simulink model "Quadcopter_Flight_Control_Simulink_payload"  (R2023b)
settings: Solver=VariableStepAuto  StartTime=0.0  StopTime=50  RelTol=1e-3
values from neighbouring files (symbols this model uses):
  A_x = 0.005581    [Quadcopter_Flight_Quantities.m]    (also in Quadcopter_Flight_Quantities_2.m)
  A_y = 0.008085    [Quadcopter_Flight_Quantities.m]    (also in Quadcopter_Flight_Quantities_2.m)
  A_z = 0.022259    [Quadcopter_Flight_Quantities.m]    (also in Quadcopter_Flight_Quantities_2.m)
  air_rho = 1.225    [Quadcopter_Flight_Quantities.m]    (also in Quadcopter_Flight_Quantities_2.m)
  Cd = 37.4    [Quadcopter_Flight_Quantities.m]    (also in Quadcopter_Flight_Quantities_2.m)
  d_p = 0.24    [Quadcopter_Flight_Quantities.m]    (also in Quadcopter_Flight_Quantities_2.m)
  g = 9.81    [Quadcopter_Flight_Quantities.m]    (also in Quadcopter_Flight_Quantities_2.m)
  k_m = 2.1783E-06    (= 2.1783e-06)    [Quadcopter_Flight_Quantities.m]    (also in Quadcopter_Flight_Quantities_2.m = 1)
  k_t = 7.3070E-05    (= 7.307e-05)    [Quadcopter_Flight_Quantities.m]    (also in Quadcopter_Flight_Quantities_2.m = 1)
  m = 2.3    [Quadcopter_Flight_Quantities.m]    (also in Quadcopter_Flight_Quantities_2.m)
  m_p = 2.530    (= 2.53)    [Quadcopter_Flight_Quantities.m]    (also in Quadcopter_Flight_Quantities_2.m)
  propeller_max = 4947*((2*pi)/60)    (= 518.048628577)    [Quadcopter_Flight_Quantities.m]    (also in Quadcopter_Flight_Quantities_2.m = 10)
libraries: matrix_library x5, slpidlib x4, aerolibasang x1, aerolibanimutils x1, shared6dof x1
settings Model: Creator=matho  LastModifiedBy=umayr
settings OptimizationCC: ReuseModelBlockBuffer=off

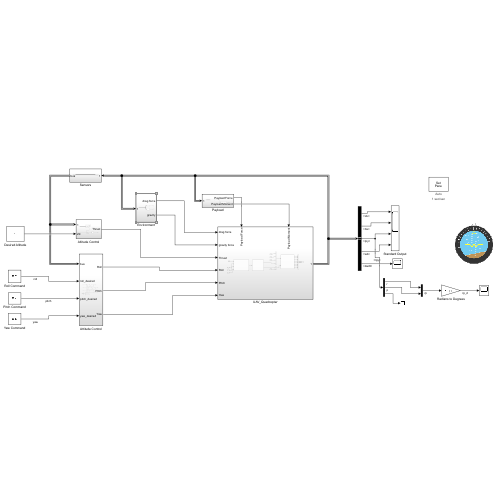
[thumbnail: Simulink's stored preview of the top-level diagram]
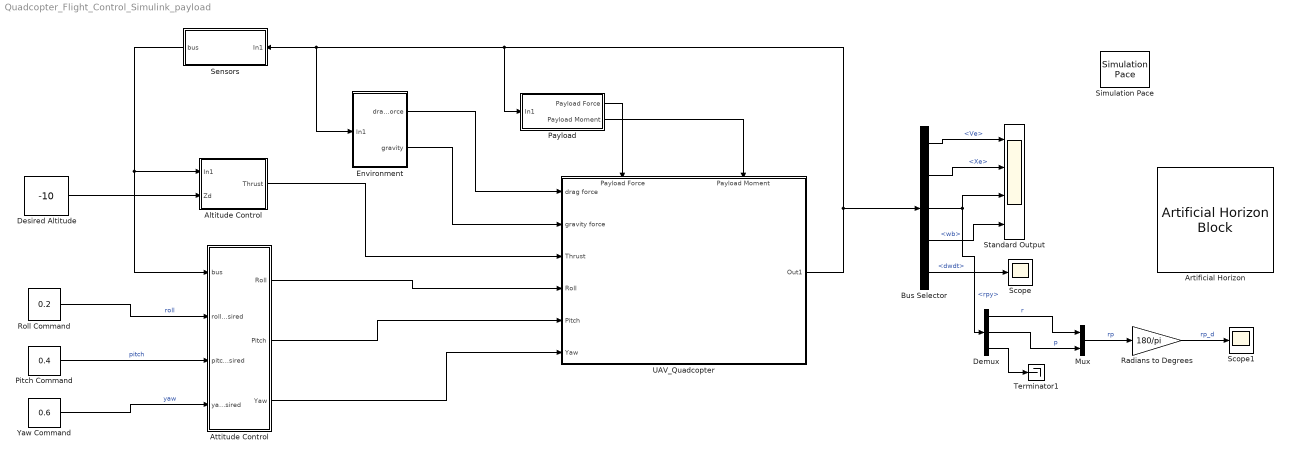
== system Quadcopter_Flight_Control_Simulink_payload ==
  Altitude Control : Subsystem
  Artificial Horizon : ArtificialHorizonBlock
  Attitude Control : Subsystem
  Bus Selector : BusSelector  OutputSignals=Ve,Xe,rpy,wb,dwdt
  Demux : Demux  Outputs=3
  Desired Altitude : Constant  Value=-10
  Environment : Subsystem
  Mux : Mux  Inputs=2
  Payload : Subsystem
  Pitch Command : Constant  Value=0.4
  Radians to Degrees : Gain  Gain=180/pi
  Roll Command : Constant  Value=0.2
  Scope : Scope
  Scope1 : Scope
  Sensors : Subsystem
  Simulation Pace : aerolibanimutils/Simulation Pace  SimulationPace=1  SleepMode=Auto  OutputPaceError=off  SampleTime=1/30
  Standard Output : Scope  NumInputPorts=4
  Terminator1 : Terminator
  UAV_Quadcopter : Subsystem
      settings: PortSchema="{\"entries\":[{\"content\":{\"sides\":[{\"content\":{\"connectorIds\":[\"In1\",\"In2\",\"In3\",\"In4\",\"In5\",\"In6\"]},\"type\":\"ConnectorPlacement.EquallySpacedRectSide\",\"uuid\":\"e9094f1d-4470-4b4b-9e27-8ba5c7ba494b\"},{\"content\":{\"connectorIds\":[\"Out1\"],\"side\":\"RIGHT\"},\"type\":\"ConnectorPlacement.EquallySpacedRectSide\",\"uuid\":\"c85a969e-3765-49d4-918f-aa5822e07523\"},{\"content\":{\"connectorIds\":[\"In7\",\"In8\"],\"side\":\"TOP\"},\"type\":\"ConnectorPlacement.EquallySpacedRectSide\",\"uuid\":\"755ec0fa-64b0-46e0-b496-7abb4caa3b84\"}]},\"type\":\"ConnectorPlacement.EquallySpacedConnector\",\"uuid\":\"b94ee3f3-a03a-4978-b802-660263939048\"}],\"packageUris\":[\"http://schema.mathworks.com/mf0/Connector/R2020b\"],\"version\":\"1.0\"}"
  Yaw Command : Constant  Value=0.6
  wires:
  Bus Selector/4 -> Standard Output/4  "<wb>"
  Bus Selector/2 -> Standard Output/2  "<Xe>"
  Bus Selector/1 -> Standard Output/1  "<Ve>"
  Sensors/1(bus) -> Altitude Control/1(In1), Attitude Control/1(bus)
  Desired Altitude/1 -> Altitude Control/2(Zd)
  Yaw Command/1 -> Attitude Control/4(yaw_desired)  "yaw"
  UAV_Quadcopter/1(Out1) -> Payload/1(In1), Environment/1(In1), Sensors/1(In1), Bus Selector/1
  Environment/1(drag force) -> UAV_Quadcopter/1(drag force)
  Environment/2(gravity) -> UAV_Quadcopter/2(gravity force)
  Altitude Control/1(Thrust) -> UAV_Quadcopter/3(Thrust)
  Attitude Control/1(Roll) -> UAV_Quadcopter/4(Roll)
  Attitude Control/2(Pitch) -> UAV_Quadcopter/5(Pitch)
  Attitude Control/3(Yaw) -> UAV_Quadcopter/6(Yaw)
  Roll Command/1 -> Attitude Control/2(roll_desired)  "roll"
  Pitch Command/1 -> Attitude Control/3(pitch_desired)  "pitch"
  Bus Selector/5 -> Scope/1  "<dwdt>"
  Payload/1(Payload Force) -> UAV_Quadcopter/7(Payload Force)
  Payload/2(Payload Moment) -> UAV_Quadcopter/8(Payload Moment)
  Radians to Degrees/1 -> Scope1/1  "rp_d"
  Demux/1 -> Mux/1  "r"
  Demux/2 -> Mux/2  "p"
  Mux/1 -> Radians to Degrees/1  "rp"
  Demux/3 -> Terminator1/1
  Bus Selector/3 -> Demux/1, Standard Output/3  "<rpy>"

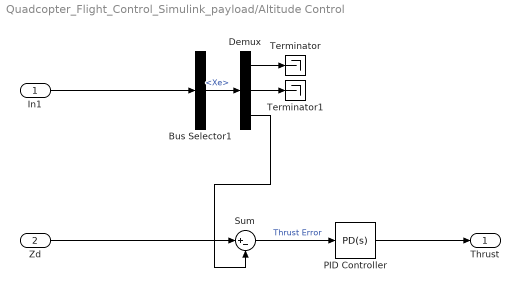
== system Quadcopter_Flight_Control_Simulink_payload/Altitude Control ==
  In1 : Inport
  Zd : Inport  Port=2
  Bus Selector1 : BusSelector  OutputSignals=Xe
  Demux : Demux  Outputs=3
  PID Controller : slpidlib/PID Controller  Controller=PD  Form=Parallel  TimeDomain=Continuous-time  UseExternalTs=off  SampleTime=-1  IntegratorMethod=Forward Euler  FilterMethod=Forward Euler  ControllerParametersSource=internal  P=5.51955288545088  I=1  UseKiTs=off  D=7.12318461741224  N=83.6239928225425  UseFilter=on  TunerSelectOption=Transfer Function Based (PID Tuner App)  InitialConditionSource=internal  InitialConditionForIntegrator=0  InitialConditionForFilter=0  DifferentiatorICPrevScaledInput=0  ExternalReset=none  TrackingMode=off  Kt=1  LimitOutput=off  SatLimitsSource=internal  UpperSaturationLimit=inf  LowerSaturationLimit=-inf  LinearizeAsGain=on  AntiWindupMode=none  Kb=1  LimitIntegrator=off  UpperIntegratorSaturationLimit=inf  LowerIntegratorSaturationLimit=-inf  POutMin=[]  POutMax=[]  IOutMin=[]  IOutMax=[]  DOutMin=[]  DOutMax=[]  NOutMin=[]  NOutMax=[]  SumOutMin=[]  SumOutMax=[]  SaturationOutMin=[]  SaturationOutMax=[]  PParamMin=[]  PParamMax=[]  IParamMin=[]  IParamMax=[]  DParamMin=[]  DParamMax=[]  NParamMin=[]  NParamMax=[]  KbParamMin=[]  KbParamMax=[]  KtParamMin=[]  KtParamMax=[]  KbOutMin=[]  KbOutMax=[]  KtOutMin=[]  KtOutMax=[]  IntegratorOutMin=[]  IntegratorOutMax=[]  FilterOutMin=[]  FilterOutMax=[]  SumI1OutMin=[]  SumI1OutMax=[]  SumI2OutMin=[]  SumI2OutMax=[]  SumI3OutMin=[]  SumI3OutMax=[]  SumI4OutMin=[]  SumI4OutMax=[]  SumDOutMin=[]  SumDOutMax=[]  DifferentiatorOutMin=[]  DifferentiatorOutMax=[]  FilterDiffOutCoefMin=[]  FilterDiffOutCoefMax=[]  ReciprocalOutMin=[]  ReciprocalOutMax=[]  SumDenOutMin=[]  SumDenOutMax=[]  SumNumOutMin=[]  SumNumOutMax=[]  DivideOutMin=[]  DivideOutMax=[]  UdiffTsProdOutMin=[]  UdiffTsProdOutMax=[]  NTsProdOutMin=[]  NTsProdOutMax=[]  UintegralTsProdOutMin=[]  UintegralTsProdOutMax=[]  UngainTsProdOutMin=[]  UngainTsProdOutMax=[]  ClampingZeroOutDataTypeStr=Inherit: Inherit via back propagation  ClampingZeroOutMin=[]  ClampingZeroOutMax=[]  FilterDenConstantOutDataTypeStr=Inherit: Inherit via back propagation  FilterDenConstantOutMin=[]  FilterDenConstantOutMax=[]  PCopyOutDataTypeStr=Inherit: Inherit via back propagation  PCopyOutMin=[]  PCopyOutMax=[]  NCopyOutDataTypeStr=Inherit: Inherit via back propagation  NCopyOutMin=[]  NCopyOutMax=[]  IntegratorContinuousStateAttributes=''  IntegratorStateMustResolveToSignalObject=off  IntegratorRTWStateStorageClass=Auto  FilterContinuousStateAttributes=''  FilterStateMustResolveToSignalObject=off  FilterRTWStateStorageClass=Auto  ParallelPVariant=InternalParameters  IdealPVariant=Disabled  IVariant=Disabled  DVariant=InternalParameters  IntegratorVariant=Disabled  SatVariant=Disabled  AWVariant=Disabled  PCopyVariant=Disabled  TRVariant=Disabled  FdbkBlocksVariant=Forward  IdealPFdbkVariant=Disabled  SatFdbkVariant=Disabled  DerivativeFilterVariant=ContFilter  NVariant=InternalParameters  NCopyVariant=Disabled  FilterICVariant=InternalICsFilter  IntegratorICVariant=Disabled  ExternalResetVariant=Disabled  TRSumVariant=Passthrough  SumFdbkVariant=Disabled  SumVariant=Sum_PD  TsampFilterVariant=InternalTs  TsampNgainVariant=Passthrough  TsampIntegralVariant=Disabled_SignalSpec  ExternalSaturationOutDataTypeStr=Inherit: Same as second input
  Sum : Sum  Inputs=|+-
  Terminator : Terminator
  Terminator1 : Terminator
  Thrust : Outport
  wires:
  Sum/1 -> PID Controller/1  "Thrust Error"
  Demux/3 -> Sum/2
  Demux/1 -> Terminator/1
  Bus Selector1/1 -> Demux/1  "<Xe>"
  Demux/2 -> Terminator1/1
  In1/1 -> Bus Selector1/1
  PID Controller/1 -> Thrust/1
  Zd/1 -> Sum/1

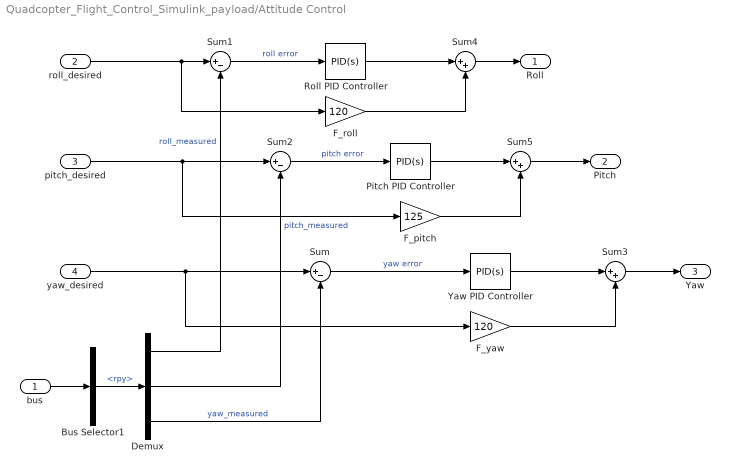
== system Quadcopter_Flight_Control_Simulink_payload/Attitude Control ==
  bus : Inport
  roll_desired : Inport  Port=2
  pitch_desired : Inport  Port=3
  yaw_desired : Inport  Port=4
  Bus Selector1 : BusSelector  OutputSignals=rpy
  Demux : Demux  Outputs=3
  F_pitch : Gain  Gain=125
  F_roll : Gain  Gain=120
  F_yaw : Gain  Gain=120
  Pitch PID Controller : slpidlib/PID Controller  Controller=PID  Form=Parallel  TimeDomain=Continuous-time  UseExternalTs=off  SampleTime=-1  IntegratorMethod=Forward Euler  FilterMethod=Forward Euler  ControllerParametersSource=internal  P=44  I=25  UseKiTs=off  D=53  N=45  UseFilter=on  TunerSelectOption=Transfer Function Based (PID Tuner App)  InitialConditionSource=internal  InitialConditionForIntegrator=0  InitialConditionForFilter=0  DifferentiatorICPrevScaledInput=0  ExternalReset=none  TrackingMode=off  Kt=1  LimitOutput=off  SatLimitsSource=internal  UpperSaturationLimit=inf  LowerSaturationLimit=-inf  LinearizeAsGain=on  AntiWindupMode=none  Kb=1  LimitIntegrator=off  UpperIntegratorSaturationLimit=inf  LowerIntegratorSaturationLimit=-inf  POutMin=[]  POutMax=[]  IOutMin=[]  IOutMax=[]  DOutMin=[]  DOutMax=[]  NOutMin=[]  NOutMax=[]  SumOutMin=[]  SumOutMax=[]  SaturationOutMin=[]  SaturationOutMax=[]  PParamMin=[]  PParamMax=[]  IParamMin=[]  IParamMax=[]  DParamMin=[]  DParamMax=[]  NParamMin=[]  NParamMax=[]  KbParamMin=[]  KbParamMax=[]  KtParamMin=[]  KtParamMax=[]  KbOutMin=[]  KbOutMax=[]  KtOutMin=[]  KtOutMax=[]  IntegratorOutMin=[]  IntegratorOutMax=[]  FilterOutMin=[]  FilterOutMax=[]  SumI1OutMin=[]  SumI1OutMax=[]  SumI2OutMin=[]  SumI2OutMax=[]  SumI3OutMin=[]  SumI3OutMax=[]  SumI4OutMin=[]  SumI4OutMax=[]  SumDOutMin=[]  SumDOutMax=[]  DifferentiatorOutMin=[]  DifferentiatorOutMax=[]  FilterDiffOutCoefMin=[]  FilterDiffOutCoefMax=[]  ReciprocalOutMin=[]  ReciprocalOutMax=[]  SumDenOutMin=[]  SumDenOutMax=[]  SumNumOutMin=[]  SumNumOutMax=[]  DivideOutMin=[]  DivideOutMax=[]  UdiffTsProdOutMin=[]  UdiffTsProdOutMax=[]  NTsProdOutMin=[]  NTsProdOutMax=[]  UintegralTsProdOutMin=[]  UintegralTsProdOutMax=[]  UngainTsProdOutMin=[]  UngainTsProdOutMax=[]  ClampingZeroOutDataTypeStr=Inherit: Inherit via back propagation  ClampingZeroOutMin=[]  ClampingZeroOutMax=[]  FilterDenConstantOutDataTypeStr=Inherit: Inherit via back propagation  FilterDenConstantOutMin=[]  FilterDenConstantOutMax=[]  PCopyOutDataTypeStr=Inherit: Inherit via back propagation  PCopyOutMin=[]  PCopyOutMax=[]  NCopyOutDataTypeStr=Inherit: Inherit via back propagation  NCopyOutMin=[]  NCopyOutMax=[]  IntegratorContinuousStateAttributes=''  IntegratorStateMustResolveToSignalObject=off  IntegratorRTWStateStorageClass=Auto  FilterContinuousStateAttributes=''  FilterStateMustResolveToSignalObject=off  FilterRTWStateStorageClass=Auto  ParallelPVariant=InternalParameters  IdealPVariant=Disabled  IVariant=InternalParameters  DVariant=InternalParameters  IntegratorVariant=Continuous  SatVariant=Disabled  AWVariant=Passthrough  PCopyVariant=Disabled  TRVariant=Disabled  FdbkBlocksVariant=Forward  IdealPFdbkVariant=Disabled  SatFdbkVariant=Disabled  DerivativeFilterVariant=ContFilter  NVariant=InternalParameters  NCopyVariant=Disabled  FilterICVariant=InternalICsFilter  IntegratorICVariant=InternalICs  ExternalResetVariant=Disabled  TRSumVariant=Passthrough  SumFdbkVariant=Disabled  SumVariant=Sum_PID  TsampFilterVariant=InternalTs  TsampNgainVariant=Passthrough  TsampIntegralVariant=Disabled_SignalSpec  ExternalSaturationOutDataTypeStr=Inherit: Same as second input
  Roll PID Controller : slpidlib/PID Controller  Controller=PID  Form=Parallel  TimeDomain=Continuous-time  UseExternalTs=off  SampleTime=-1  IntegratorMethod=Forward Euler  FilterMethod=Forward Euler  ControllerParametersSource=internal  P=42  I=24  UseKiTs=off  D=48  N=45  UseFilter=on  TunerSelectOption=Transfer Function Based (PID Tuner App)  InitialConditionSource=internal  InitialConditionForIntegrator=0  InitialConditionForFilter=0  DifferentiatorICPrevScaledInput=0  ExternalReset=none  TrackingMode=off  Kt=1  LimitOutput=off  SatLimitsSource=internal  UpperSaturationLimit=inf  LowerSaturationLimit=-inf  LinearizeAsGain=on  AntiWindupMode=none  Kb=1  LimitIntegrator=off  UpperIntegratorSaturationLimit=inf  LowerIntegratorSaturationLimit=-inf  POutMin=[]  POutMax=[]  IOutMin=[]  IOutMax=[]  DOutMin=[]  DOutMax=[]  NOutMin=[]  NOutMax=[]  SumOutMin=[]  SumOutMax=[]  SaturationOutMin=[]  SaturationOutMax=[]  PParamMin=[]  PParamMax=[]  IParamMin=[]  IParamMax=[]  DParamMin=[]  DParamMax=[]  NParamMin=[]  NParamMax=[]  KbParamMin=[]  KbParamMax=[]  KtParamMin=[]  KtParamMax=[]  KbOutMin=[]  KbOutMax=[]  KtOutMin=[]  KtOutMax=[]  IntegratorOutMin=[]  IntegratorOutMax=[]  FilterOutMin=[]  FilterOutMax=[]  SumI1OutMin=[]  SumI1OutMax=[]  SumI2OutMin=[]  SumI2OutMax=[]  SumI3OutMin=[]  SumI3OutMax=[]  SumI4OutMin=[]  SumI4OutMax=[]  SumDOutMin=[]  SumDOutMax=[]  DifferentiatorOutMin=[]  DifferentiatorOutMax=[]  FilterDiffOutCoefMin=[]  FilterDiffOutCoefMax=[]  ReciprocalOutMin=[]  ReciprocalOutMax=[]  SumDenOutMin=[]  SumDenOutMax=[]  SumNumOutMin=[]  SumNumOutMax=[]  DivideOutMin=[]  DivideOutMax=[]  UdiffTsProdOutMin=[]  UdiffTsProdOutMax=[]  NTsProdOutMin=[]  NTsProdOutMax=[]  UintegralTsProdOutMin=[]  UintegralTsProdOutMax=[]  UngainTsProdOutMin=[]  UngainTsProdOutMax=[]  ClampingZeroOutDataTypeStr=Inherit: Inherit via back propagation  ClampingZeroOutMin=[]  ClampingZeroOutMax=[]  FilterDenConstantOutDataTypeStr=Inherit: Inherit via back propagation  FilterDenConstantOutMin=[]  FilterDenConstantOutMax=[]  PCopyOutDataTypeStr=Inherit: Inherit via back propagation  PCopyOutMin=[]  PCopyOutMax=[]  NCopyOutDataTypeStr=Inherit: Inherit via back propagation  NCopyOutMin=[]  NCopyOutMax=[]  IntegratorContinuousStateAttributes=''  IntegratorStateMustResolveToSignalObject=off  IntegratorRTWStateStorageClass=Auto  FilterContinuousStateAttributes=''  FilterStateMustResolveToSignalObject=off  FilterRTWStateStorageClass=Auto  ParallelPVariant=InternalParameters  IdealPVariant=Disabled  IVariant=InternalParameters  DVariant=InternalParameters  IntegratorVariant=Continuous  SatVariant=Disabled  AWVariant=Passthrough  PCopyVariant=Disabled  TRVariant=Disabled  FdbkBlocksVariant=Forward  IdealPFdbkVariant=Disabled  SatFdbkVariant=Disabled  DerivativeFilterVariant=ContFilter  NVariant=InternalParameters  NCopyVariant=Disabled  FilterICVariant=InternalICsFilter  IntegratorICVariant=InternalICs  ExternalResetVariant=Disabled  TRSumVariant=Passthrough  SumFdbkVariant=Disabled  SumVariant=Sum_PID  TsampFilterVariant=InternalTs  TsampNgainVariant=Passthrough  TsampIntegralVariant=Disabled_SignalSpec  ExternalSaturationOutDataTypeStr=Inherit: Same as second input
  Sum : Sum  Inputs=|+-
  Sum1 : Sum  Inputs=|+-
  Sum2 : Sum  Inputs=|+-
  Sum3 : Sum  Inputs=|++
  Sum4 : Sum  Inputs=|++
  Sum5 : Sum  Inputs=|++
  Yaw PID Controller : slpidlib/PID Controller  Controller=PID  Form=Parallel  TimeDomain=Continuous-time  UseExternalTs=off  SampleTime=-1  IntegratorMethod=Forward Euler  FilterMethod=Forward Euler  ControllerParametersSource=internal  P=42  I=28  UseKiTs=off  D=48  N=45  UseFilter=on  TunerSelectOption=Transfer Function Based (PID Tuner App)  InitialConditionSource=internal  InitialConditionForIntegrator=0  InitialConditionForFilter=0  DifferentiatorICPrevScaledInput=0  ExternalReset=none  TrackingMode=off  Kt=1  LimitOutput=off  SatLimitsSource=internal  UpperSaturationLimit=inf  LowerSaturationLimit=-inf  LinearizeAsGain=on  AntiWindupMode=none  Kb=1  LimitIntegrator=off  UpperIntegratorSaturationLimit=inf  LowerIntegratorSaturationLimit=-inf  POutMin=[]  POutMax=[]  IOutMin=[]  IOutMax=[]  DOutMin=[]  DOutMax=[]  NOutMin=[]  NOutMax=[]  SumOutMin=[]  SumOutMax=[]  SaturationOutMin=[]  SaturationOutMax=[]  PParamMin=[]  PParamMax=[]  IParamMin=[]  IParamMax=[]  DParamMin=[]  DParamMax=[]  NParamMin=[]  NParamMax=[]  KbParamMin=[]  KbParamMax=[]  KtParamMin=[]  KtParamMax=[]  KbOutMin=[]  KbOutMax=[]  KtOutMin=[]  KtOutMax=[]  IntegratorOutMin=[]  IntegratorOutMax=[]  FilterOutMin=[]  FilterOutMax=[]  SumI1OutMin=[]  SumI1OutMax=[]  SumI2OutMin=[]  SumI2OutMax=[]  SumI3OutMin=[]  SumI3OutMax=[]  SumI4OutMin=[]  SumI4OutMax=[]  SumDOutMin=[]  SumDOutMax=[]  DifferentiatorOutMin=[]  DifferentiatorOutMax=[]  FilterDiffOutCoefMin=[]  FilterDiffOutCoefMax=[]  ReciprocalOutMin=[]  ReciprocalOutMax=[]  SumDenOutMin=[]  SumDenOutMax=[]  SumNumOutMin=[]  SumNumOutMax=[]  DivideOutMin=[]  DivideOutMax=[]  UdiffTsProdOutMin=[]  UdiffTsProdOutMax=[]  NTsProdOutMin=[]  NTsProdOutMax=[]  UintegralTsProdOutMin=[]  UintegralTsProdOutMax=[]  UngainTsProdOutMin=[]  UngainTsProdOutMax=[]  ClampingZeroOutDataTypeStr=Inherit: Inherit via back propagation  ClampingZeroOutMin=[]  ClampingZeroOutMax=[]  FilterDenConstantOutDataTypeStr=Inherit: Inherit via back propagation  FilterDenConstantOutMin=[]  FilterDenConstantOutMax=[]  PCopyOutDataTypeStr=Inherit: Inherit via back propagation  PCopyOutMin=[]  PCopyOutMax=[]  NCopyOutDataTypeStr=Inherit: Inherit via back propagation  NCopyOutMin=[]  NCopyOutMax=[]  IntegratorContinuousStateAttributes=''  IntegratorStateMustResolveToSignalObject=off  IntegratorRTWStateStorageClass=Auto  FilterContinuousStateAttributes=''  FilterStateMustResolveToSignalObject=off  FilterRTWStateStorageClass=Auto  ParallelPVariant=InternalParameters  IdealPVariant=Disabled  IVariant=InternalParameters  DVariant=InternalParameters  IntegratorVariant=Continuous  SatVariant=Disabled  AWVariant=Passthrough  PCopyVariant=Disabled  TRVariant=Disabled  FdbkBlocksVariant=Forward  IdealPFdbkVariant=Disabled  SatFdbkVariant=Disabled  DerivativeFilterVariant=ContFilter  NVariant=InternalParameters  NCopyVariant=Disabled  FilterICVariant=InternalICsFilter  IntegratorICVariant=InternalICs  ExternalResetVariant=Disabled  TRSumVariant=Passthrough  SumFdbkVariant=Disabled  SumVariant=Sum_PID  TsampFilterVariant=InternalTs  TsampNgainVariant=Passthrough  TsampIntegralVariant=Disabled_SignalSpec  ExternalSaturationOutDataTypeStr=Inherit: Same as second input
  Roll : Outport
  Pitch : Outport  Port=2
  Yaw : Outport  Port=3
  wires:
  yaw_desired/1 -> Sum/1, F_yaw/1
  Demux/3 -> Sum/2  "yaw_measured"
  Demux/2 -> Sum2/2  "pitch_measured"
  Demux/1 -> Sum1/2  "roll_measured"
  Bus Selector1/1 -> Demux/1  "<rpy>"
  bus/1 -> Bus Selector1/1
  roll_desired/1 -> F_roll/1, Sum1/1
  pitch_desired/1 -> F_pitch/1, Sum2/1
  Sum1/1 -> Roll PID Controller/1  "roll error"
  Sum2/1 -> Pitch PID Controller/1  "pitch error"
  Pitch PID Controller/1 -> Sum5/1
  Roll PID Controller/1 -> Sum4/1
  Sum/1 -> Yaw PID Controller/1  "yaw error"
  Yaw PID Controller/1 -> Sum3/1
  F_yaw/1 -> Sum3/2
  Sum3/1 -> Yaw/1
  F_roll/1 -> Sum4/2
  Sum4/1 -> Roll/1
  F_pitch/1 -> Sum5/2
  Sum5/1 -> Pitch/1

== system Quadcopter_Flight_Control_Simulink_payload/Environment ==
  In1 : Inport
  Aerodynamic Drag : Subsystem
  Gravitational Force : Subsystem
  drag force : Outport
  gravity : Outport  Port=2
  wires:
  In1/1 -> Aerodynamic Drag/1(In2), Gravitational Force/1(In1)
  Aerodynamic Drag/1(Drag) -> drag force/1
  Gravitational Force/1(Out1) -> gravity/1

== system Quadcopter_Flight_Control_Simulink_payload/Payload ==
  In1 : Inport
  Force : Subsystem
  Moment : Subsystem
  Payload Force : Outport
  Payload Moment : Outport  Port=2
  wires:
  In1/1 -> Force/1(In1)
  Force/1(Payload Weight) -> Payload Force/1, Moment/1(Payload Force)
  Moment/1(Payload Moment) -> Payload Moment/1

== system Quadcopter_Flight_Control_Simulink_payload/Sensors ==
  In1 : Inport
  bus : Outport
  wires:
  In1/1 -> bus/1

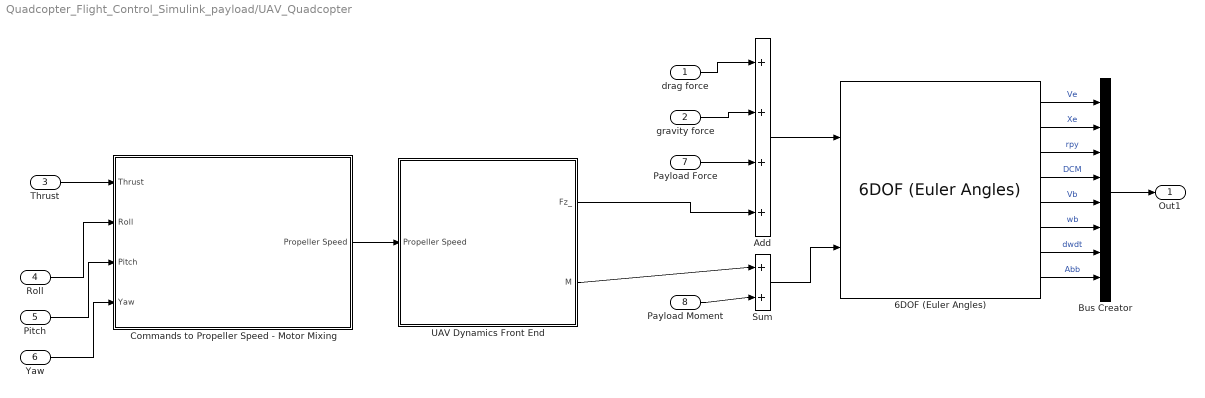
== system Quadcopter_Flight_Control_Simulink_payload/UAV_Quadcopter ==
  drag force : Inport
  gravity force : Inport  Port=2
  Thrust : Inport  Port=3
  Roll : Inport  Port=4
  Pitch : Inport  Port=5
  Yaw : Inport  Port=6
  Payload Force : Inport  Port=7
  Payload Moment : Inport  Port=8
  6DOF (Euler Angles) : shared6dof/6DOF (Euler Angles)  units=Metric (MKS)  mtype=Fixed  rep=Euler Angles  xme_0=[0 0 0]  Vm_0=[0 0 0]  eul_0=[0 0 0]  pm_0=[0 0 0]  mass_0=1.0  mass_e=0.5  mass_f=2.0  inertia=eye(3)  inertia_e=eye(3)  inertia_f=2*eye(3)  k_quat=1.0  vre_flag=on  abi_flag=off  aMode=0  xme_statename=''  Vm_statename=''  eul_statename=''  quat_statename=''  pm_statename=''  mass_statename=''
  Add : Sum  Inputs=++++
  Bus Creator : BusCreator  Inputs=8
  "Commands to Propeller Speed - Motor Mixing " : Subsystem
  Sum : Sum  Inputs=|++
  UAV Dynamics Front End : Subsystem
  Out1 : Outport
  wires:
  Bus Creator/1 -> Out1/1
  UAV Dynamics Front End/2(M) -> Sum/1
  "Commands to Propeller Speed - Motor Mixing "/1(Propeller Speed) -> UAV Dynamics Front End/1(Propeller Speed)
  6DOF (Euler Angles)/1 -> Bus Creator/1  "Ve"
  6DOF (Euler Angles)/8 -> Bus Creator/8  "Abb"
  Add/1 -> 6DOF (Euler Angles)/1
  6DOF (Euler Angles)/3 -> Bus Creator/3  "rpy"
  6DOF (Euler Angles)/7 -> Bus Creator/7  "dwdt"
  6DOF (Euler Angles)/2 -> Bus Creator/2  "Xe"
  6DOF (Euler Angles)/4 -> Bus Creator/4  "DCM"
  6DOF (Euler Angles)/5 -> Bus Creator/5  "Vb"
  6DOF (Euler Angles)/6 -> Bus Creator/6  "wb"
  UAV Dynamics Front End/1(Fz_) -> Add/4
  gravity force/1 -> Add/2
  drag force/1 -> Add/1
  Thrust/1 -> "Commands to Propeller Speed - Motor Mixing "/1(Thrust)
  Yaw/1 -> "Commands to Propeller Speed - Motor Mixing "/4(Yaw)
  Pitch/1 -> "Commands to Propeller Speed - Motor Mixing "/3(Pitch)
  Roll/1 -> "Commands to Propeller Speed - Motor Mixing "/2(Roll)
  Payload Force/1 -> Add/3
  Payload Moment/1 -> Sum/2
  Sum/1 -> 6DOF (Euler Angles)/2

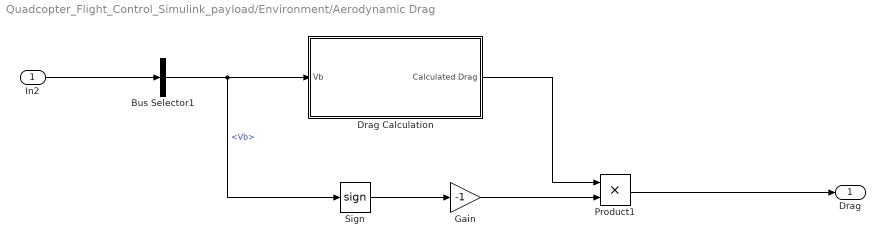
== system Quadcopter_Flight_Control_Simulink_payload/Environment/Aerodynamic Drag ==
  In2 : Inport
  Bus Selector1 : BusSelector  OutputSignals=Vb
  Drag Calculation : Subsystem
  Gain : Gain  Gain=-1
  Product1 : Product
  Sign : Signum  ZeroCross=off
  Drag : Outport
  wires:
  In2/1 -> Bus Selector1/1
  Product1/1 -> Drag/1
  Bus Selector1/1 -> Sign/1, Drag Calculation/1(Vb)  "<Vb>"
  Sign/1 -> Gain/1
  Gain/1 -> Product1/2
  Drag Calculation/1(Calculated Drag) -> Product1/1

== system Quadcopter_Flight_Control_Simulink_payload/Environment/Gravitational Force ==
  In1 : Inport
  Gravitational Accl : Subsystem
  Mass : Gain  Gain=m
  Out1 : Outport
  wires:
  Mass/1 -> Out1/1
  Gravitational Accl/1(Out1) -> Mass/1
  In1/1 -> Gravitational Accl/1(In1)

== system Quadcopter_Flight_Control_Simulink_payload/Payload/Force ==
  In1 : Inport
  Gravitational Accl : Subsystem
  Mass of Payload : Gain  Gain=m_p
  Payload Weight : Outport
  wires:
  In1/1 -> Gravitational Accl/1(In1)
  Gravitational Accl/1(Out1) -> Mass of Payload/1
  Mass of Payload/1 -> Payload Weight/1

== system Quadcopter_Flight_Control_Simulink_payload/Payload/Moment ==
  Payload Force : Inport
  Cross Product : matrix_library/Cross Product
  Payload Position : Constant  Value=[0;0;d_p]
  Payload Moment : Outport
  wires:
  Payload Force/1 -> Cross Product/2
  Payload Position/1 -> Cross Product/1
  Cross Product/1 -> Payload Moment/1

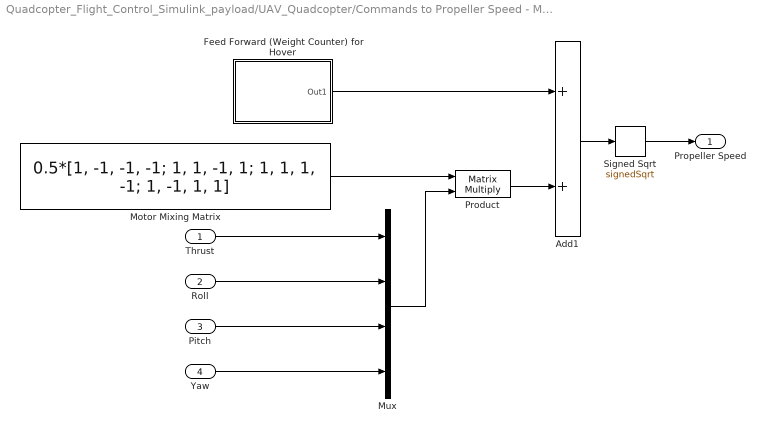
== system Quadcopter_Flight_Control_Simulink_payload/UAV_Quadcopter/Commands to Propeller Speed - Motor Mixing  ==
  Thrust : Inport
  Roll : Inport  Port=2
  Pitch : Inport  Port=3
  Yaw : Inport  Port=4
  Add1 : Sum
  Feed Forward (Weight Counter) for Hover : Subsystem
  Motor Mixing Matrix : Constant  Value=0.5*[1, -1, -1, -1; 1, 1, -1, 1; 1, 1, 1, -1; 1, -1, 1, 1]  VectorParams1D=off
  Mux : Mux
  Product : Product  Multiplication=Matrix(*)
  Signed Sqrt : Sqrt  Operator=signedSqrt
  Propeller Speed : Outport
  wires:
  Feed Forward (Weight Counter) for Hover/1(Out1) -> Add1/1
  Mux/1 -> Product/2
  Pitch/1 -> Mux/3
  Product/1 -> Add1/2
  Roll/1 -> Mux/2
  Motor Mixing Matrix/1 -> Product/1
  Yaw/1 -> Mux/4
  Thrust/1 -> Mux/1
  Add1/1 -> Signed Sqrt/1
  Signed Sqrt/1 -> Propeller Speed/1

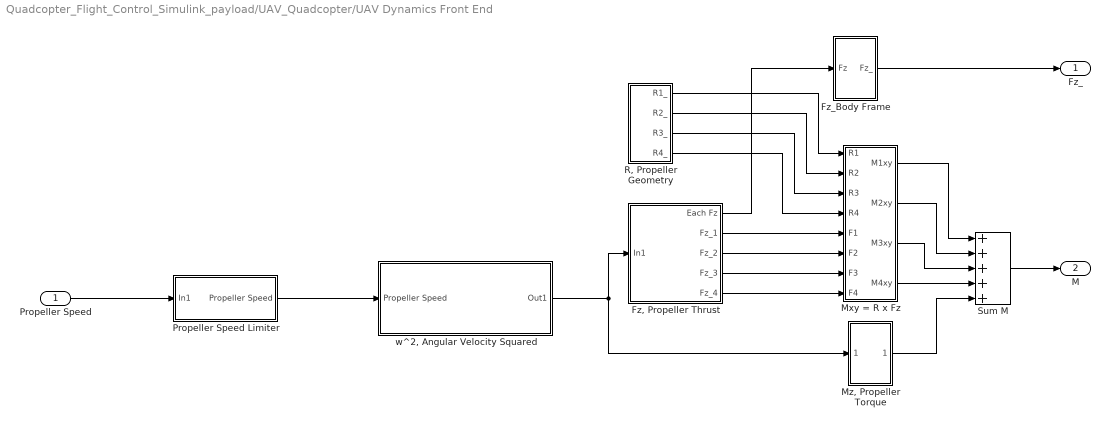
== system Quadcopter_Flight_Control_Simulink_payload/UAV_Quadcopter/UAV Dynamics Front End ==
  Propeller Speed : Inport
  "Fz, Propeller Thrust" : Subsystem
  Fz_Body Frame : Subsystem
  Mxy = R x Fz : Subsystem
  "Mz, Propeller Torque " : Subsystem
  Propeller Speed Limiter : Subsystem
  "R, Propeller Geometry" : Subsystem
  Sum M : Sum  Inputs=+++++
  "w^2, Angular Velocity Squared" : Subsystem
  Fz_ : Outport
  M : Outport  Port=2
  wires:
  "Fz, Propeller Thrust"/4(Fz_3) -> Mxy = R x Fz/7(F3)
  "Fz, Propeller Thrust"/2(Fz_1) -> Mxy = R x Fz/5(F1)
  Mxy = R x Fz/4(M4xy) -> Sum M/4
  "R, Propeller Geometry"/2(R2_) -> Mxy = R x Fz/2(R2)
  "Fz, Propeller Thrust"/5(Fz_4) -> Mxy = R x Fz/8(F4)
  Mxy = R x Fz/2(M2xy) -> Sum M/2
  "Fz, Propeller Thrust"/3(Fz_2) -> Mxy = R x Fz/6(F2)
  "R, Propeller Geometry"/3(R3_) -> Mxy = R x Fz/3(R3)
  "R, Propeller Geometry"/4(R4_) -> Mxy = R x Fz/4(R4)
  Propeller Speed/1 -> Propeller Speed Limiter/1(In1)
  Mxy = R x Fz/3(M3xy) -> Sum M/3
  "Fz, Propeller Thrust"/1(Each Fz) -> Fz_Body Frame/1(Fz)
  "w^2, Angular Velocity Squared"/1(Out1) -> "Mz, Propeller Torque "/1(In1), "Fz, Propeller Thrust"/1(In1)
  "Mz, Propeller Torque "/1(Out1) -> Sum M/5
  Mxy = R x Fz/1(M1xy) -> Sum M/1
  "R, Propeller Geometry"/1(R1_) -> Mxy = R x Fz/1(R1)
  Sum M/1 -> M/1
  Fz_Body Frame/1(Fz_) -> Fz_/1
  Propeller Speed Limiter/1(Propeller Speed) -> "w^2, Angular Velocity Squared"/1(Propeller Speed)

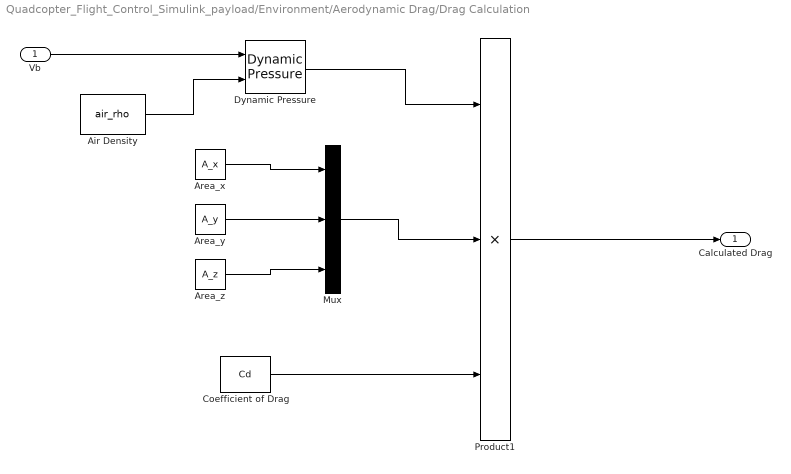
== system Quadcopter_Flight_Control_Simulink_payload/Environment/Aerodynamic Drag/Drag Calculation ==
  Vb : Inport
  Air Density : Constant  Value=air_rho
  Area_x : Constant  Value=A_x
  Area_y : Constant  Value=A_y
  Area_z : Constant  Value=A_z
  Coefficient of Drag : Constant  Value=Cd
  Dynamic Pressure : aerolibasang/Dynamic Pressure
  Mux : Mux  Inputs=3
  Product1 : Product  Inputs=3
  Calculated Drag : Outport
  wires:
  Mux/1 -> Product1/2
  Area_x/1 -> Mux/1
  Vb/1 -> Dynamic Pressure/1
  Area_z/1 -> Mux/3
  Area_y/1 -> Mux/2
  Dynamic Pressure/1 -> Product1/1
  Coefficient of Drag/1 -> Product1/3
  Air Density/1 -> Dynamic Pressure/2
  Product1/1 -> Calculated Drag/1

== system Quadcopter_Flight_Control_Simulink_payload/Environment/Gravitational Force/Gravitational Accl ==
  In1 : Inport
  Bus Selector : BusSelector  OutputSignals=DCM
  Constant : Constant  Value=[0;0;g]
  Product : Product  Multiplication=Matrix(*)
  Out1 : Outport
  wires:
  Constant/1 -> Product/2
  In1/1 -> Bus Selector/1
  Product/1 -> Out1/1
  Bus Selector/1 -> Product/1  "<DCM>"

== system Quadcopter_Flight_Control_Simulink_payload/Payload/Force/Gravitational Accl ==
  In1 : Inport
  Bus Selector : BusSelector  OutputSignals=DCM
  Constant : Constant  Value=[0;0;g]
  Product : Product  Multiplication=Matrix(*)
  Out1 : Outport
  wires:
  Constant/1 -> Product/2
  In1/1 -> Bus Selector/1
  Product/1 -> Out1/1
  Bus Selector/1 -> Product/1  "<DCM>"

== system Quadcopter_Flight_Control_Simulink_payload/UAV_Quadcopter/Commands to Propeller Speed - Motor Mixing /Feed Forward (Weight Counter) for Hover ==
  Constant1 : Constant  Value=[1;1;1;1]
  Conversion Coefficient : Gain  Gain=g/4
  Direction : Gain  Gain=-1
  Mass of Drone : Gain  Gain=m
  Out1 : Outport
  wires:
  Constant1/1 -> Mass of Drone/1
  Direction/1 -> Conversion Coefficient/1
  Mass of Drone/1 -> Direction/1
  Conversion Coefficient/1 -> Out1/1

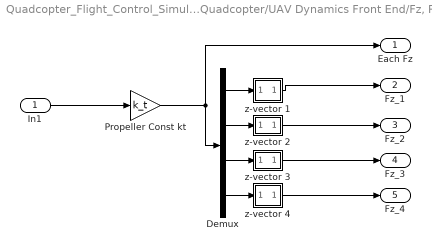
== system Quadcopter_Flight_Control_Simulink_payload/UAV_Quadcopter/UAV Dynamics Front End/Fz, Propeller Thrust ==
  In1 : Inport
  Demux : Demux
  Propeller Const kt : Gain  Gain=k_t
  z-vector 1 : Subsystem
  z-vector 2 : Subsystem
  z-vector 3 : Subsystem
  z-vector 4 : Subsystem
  Each Fz : Outport
  Fz_1 : Outport  Port=2
  Fz_2 : Outport  Port=3
  Fz_3 : Outport  Port=4
  Fz_4 : Outport  Port=5
  wires:
  Demux/4 -> z-vector 4/1(In1)
  Demux/1 -> z-vector 1/1(In1)
  z-vector 3/1(Out1) -> Fz_3/1
  z-vector 2/1(Out1) -> Fz_2/1
  Propeller Const kt/1 -> Each Fz/1, Demux/1
  z-vector 1/1(Out1) -> Fz_1/1
  Demux/2 -> z-vector 2/1(In1)
  Demux/3 -> z-vector 3/1(In1)
  z-vector 4/1(Out1) -> Fz_4/1
  In1/1 -> Propeller Const kt/1

== system Quadcopter_Flight_Control_Simulink_payload/UAV_Quadcopter/UAV Dynamics Front End/Fz_Body Frame ==
  Fz : Inport
  Sum of Elements : Sum  Inputs=+
  "z-vector " : Subsystem
  Fz_ : Outport
  wires:
  Sum of Elements/1 -> "z-vector "/1(Fz_in)
  "z-vector "/1(Fz_out) -> Fz_/1
  Fz/1 -> Sum of Elements/1

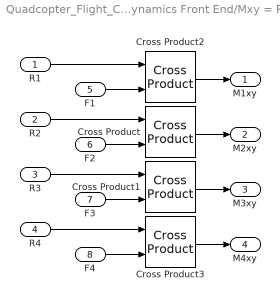
== system Quadcopter_Flight_Control_Simulink_payload/UAV_Quadcopter/UAV Dynamics Front End/Mxy = R x Fz ==
  R1 : Inport
  R2 : Inport  Port=2
  R3 : Inport  Port=3
  R4 : Inport  Port=4
  F1 : Inport  Port=5
  F2 : Inport  Port=6
  F3 : Inport  Port=7
  F4 : Inport  Port=8
  Cross Product{,1..3} (4 alike) : matrix_library/Cross Product
  M1xy : Outport
  M2xy : Outport  Port=2
  M3xy : Outport  Port=3
  M4xy : Outport  Port=4
  wires:
  F4/1 -> Cross Product3/2
  Cross Product/1 -> M2xy/1
  Cross Product2/1 -> M1xy/1
  F1/1 -> Cross Product2/2
  R2/1 -> Cross Product/1
  F3/1 -> Cross Product1/2
  Cross Product3/1 -> M4xy/1
  Cross Product1/1 -> M3xy/1
  F2/1 -> Cross Product/2
  R3/1 -> Cross Product1/1
  R1/1 -> Cross Product2/1
  R4/1 -> Cross Product3/1

== system Quadcopter_Flight_Control_Simulink_payload/UAV_Quadcopter/UAV Dynamics Front End/Mz, Propeller Torque  ==
  In1 : Inport
  "Motor Torque Constant, km" : Gain  Gain=k_m
  z-torque : Subsystem
  z-vector 5 : Subsystem
  Out1 : Outport
  wires:
  z-torque/1(Out1) -> z-vector 5/1(In1)
  "Motor Torque Constant, km"/1 -> z-torque/1(In1)
  z-vector 5/1(Out1) -> Out1/1
  In1/1 -> "Motor Torque Constant, km"/1

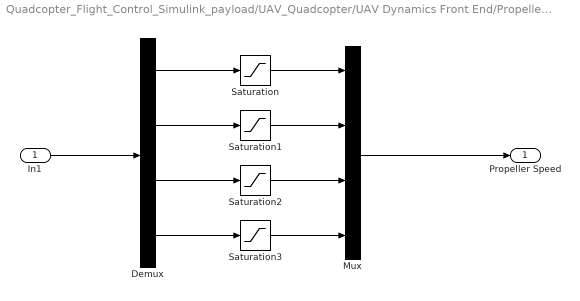
== system Quadcopter_Flight_Control_Simulink_payload/UAV_Quadcopter/UAV Dynamics Front End/Propeller Speed Limiter ==
  In1 : Inport
  Demux : Demux
  Mux : Mux
  Saturation{,1..3} (4 alike) : Saturate  UpperLimit=0  LowerLimit=-propeller_max
  Propeller Speed : Outport
  wires:
  In1/1 -> Demux/1
  Demux/1 -> Saturation/1
  Demux/2 -> Saturation1/1
  Demux/3 -> Saturation2/1
  Demux/4 -> Saturation3/1
  Saturation/1 -> Mux/1
  Saturation1/1 -> Mux/2
  Saturation2/1 -> Mux/3
  Saturation3/1 -> Mux/4
  Mux/1 -> Propeller Speed/1

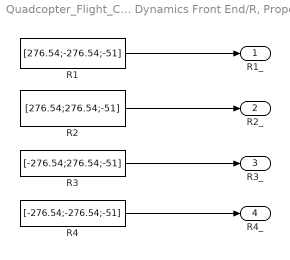
== system Quadcopter_Flight_Control_Simulink_payload/UAV_Quadcopter/UAV Dynamics Front End/R, Propeller Geometry ==
  R1 : Constant  Value=[276.54;-276.54;-51]
  R2 : Constant  Value=[276.54;276.54;-51]
  R3 : Constant  Value=[-276.54;276.54;-51]
  R4 : Constant  Value=[-276.54;-276.54;-51]
  R1_ : Outport
  R2_ : Outport  Port=2
  R3_ : Outport  Port=3
  R4_ : Outport  Port=4
  wires:
  R1/1 -> R1_/1
  R4/1 -> R4_/1
  R3/1 -> R3_/1
  R2/1 -> R2_/1

== system Quadcopter_Flight_Control_Simulink_payload/UAV_Quadcopter/UAV Dynamics Front End/w^2, Angular Velocity Squared ==
  Propeller Speed : Inport
  Abs : Abs  SaturateOnIntegerOverflow=off
  Product : Product
  Out1 : Outport
  wires:
  Propeller Speed/1 -> Product/2, Abs/1
  Abs/1 -> Product/1
  Product/1 -> Out1/1

== system Quadcopter_Flight_Control_Simulink_payload/UAV_Quadcopter/UAV Dynamics Front End/Fz, Propeller Thrust/z-vector 1 ==
  In1 : Inport
  Divide : Product  Inputs=**
  az : Constant  Value=[0;0;1]
  Out1 : Outport
  wires:
  az/1 -> Divide/1
  Divide/1 -> Out1/1
  In1/1 -> Divide/2

== system Quadcopter_Flight_Control_Simulink_payload/UAV_Quadcopter/UAV Dynamics Front End/Fz, Propeller Thrust/z-vector 2 ==
  In1 : Inport
  Divide : Product  Inputs=**
  az : Constant  Value=[0;0;1]
  Out1 : Outport
  wires:
  az/1 -> Divide/1
  Divide/1 -> Out1/1
  In1/1 -> Divide/2

== system Quadcopter_Flight_Control_Simulink_payload/UAV_Quadcopter/UAV Dynamics Front End/Fz, Propeller Thrust/z-vector 3 ==
  In1 : Inport
  Divide : Product  Inputs=**
  az : Constant  Value=[0;0;1]
  Out1 : Outport
  wires:
  az/1 -> Divide/1
  Divide/1 -> Out1/1
  In1/1 -> Divide/2

== system Quadcopter_Flight_Control_Simulink_payload/UAV_Quadcopter/UAV Dynamics Front End/Fz, Propeller Thrust/z-vector 4 ==
  In1 : Inport
  Divide : Product  Inputs=**
  az : Constant  Value=[0;0;1]
  Out1 : Outport
  wires:
  az/1 -> Divide/1
  Divide/1 -> Out1/1
  In1/1 -> Divide/2

== system Quadcopter_Flight_Control_Simulink_payload/UAV_Quadcopter/UAV Dynamics Front End/Fz_Body Frame/z-vector  ==
  Fz_in : Inport
  Divide : Product  Inputs=**
  az : Constant  Value=[0;0;1]
  Fz_out : Outport
  wires:
  az/1 -> Divide/1
  Divide/1 -> Fz_out/1
  Fz_in/1 -> Divide/2

== system Quadcopter_Flight_Control_Simulink_payload/UAV_Quadcopter/UAV Dynamics Front End/Mz, Propeller Torque /z-torque ==
  In1 : Inport
  Constant : Constant  Value=[-1; 1; -1; 1]
  Product1 : Product
  Sum of Elements : Sum  Inputs=+
  Out1 : Outport
  wires:
  Constant/1 -> Product1/1
  In1/1 -> Product1/2
  Product1/1 -> Sum of Elements/1
  Sum of Elements/1 -> Out1/1

== system Quadcopter_Flight_Control_Simulink_payload/UAV_Quadcopter/UAV Dynamics Front End/Mz, Propeller Torque /z-vector 5 ==
  In1 : Inport
  Divide : Product  Inputs=**
  az : Constant  Value=[0;0;1]
  Out1 : Outport
  wires:
  az/1 -> Divide/1
  Divide/1 -> Out1/1
  In1/1 -> Divide/2
